simulink model "FBFunctions_Athira"  (R2018b)
settings: Solver=VariableStepAuto  StartTime=0.0  StopTime=10.0  RelTol=1e-3
values from neighbouring files (symbols this model uses):
  DIV = int32(25)    [setup.m]
  fractionalNumBits = 24    [setup.m]
  integerNumBits = 32    [setup.m]
  SUB = int32(23)    [setup.m]
undefined symbols (not defined in the file or in its folder): mask
libraries: library x94, hdlsllib x21, simulink x2
settings Model: Creator=hiterd  LastModifiedBy=jayakumarav
settings SFSimCC: SimUseLocalCustomCode=off
settings RTWCC: RTWUseLocalCustomCode=off

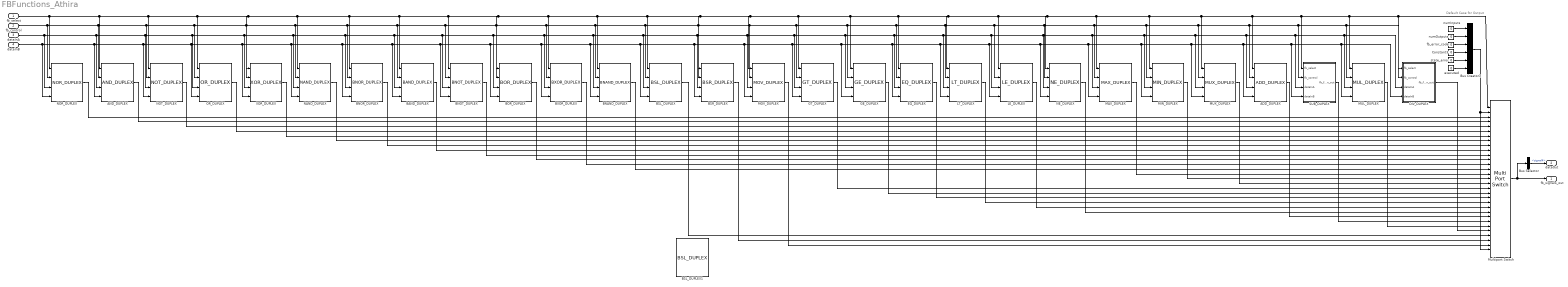
== system FBFunctions_Athira ==
  note: Default Case for Output
  fb_select : Inport  OutDataTypeStr=int32
  fb_control : Inport  Port=2  OutDataTypeStr=Bus: fb_control
  dataInA : Inport  Port=3  OutDataTypeStr=int32
  dataInB : Inport  Port=4  OutDataTypeStr=int32
  ADD_DUPLEX : library/ADD_DUPLEX  SystemSampleTime=-1  VariantControl=MUX_FB
  AND_DUPLEX : library/AND_DUPLEX  SystemSampleTime=-1  VariantControl=MUX_FB
  BAND_DUPLEX : library/BAND_DUPLEX  SystemSampleTime=-1  VariantControl=MUX_FB
  BNAND_DUPLEX : library/BNAND_DUPLEX  SystemSampleTime=-1  VariantControl=MUX_FB
  BNOR_DUPLEX : library/BNOR_DUPLEX  SystemSampleTime=-1  VariantControl=MUX_FB
  BNOT_DUPLEX : library/BNOT_DUPLEX  SystemSampleTime=-1  VariantControl=MUX_FB
  BOR_DUPLEX : library/BOR_DUPLEX  SystemSampleTime=-1  VariantControl=MUX_FB
  BSL_DUPLEX : library/BSL_DUPLEX  SystemSampleTime=-1  VariantControl=MUX_FB
  BSL_DUPLEX1 : library/BSL_DUPLEX  SystemSampleTime=-1  VariantControl=MUX_FB
  BSR_DUPLEX : library/BSR_DUPLEX  SystemSampleTime=-1  VariantControl=MUX_FB
  BXOR_DUPLEX : library/BXOR_DUPLEX  SystemSampleTime=-1  VariantControl=MUX_FB
  Bus Creator1 : BusCreator  Inputs=6  OutDataTypeStr=Bus: fb_functions_out
  Bus Selector : BusSelector  OutputSignals=signal4
  Constant3 : Constant  Value=0  OutDataTypeStr=int32  SampleTime=-1
  DIV_DUPLEX : Subsystem  AncestorBlock=library/DIV_DUPLEX  TreatAsAtomicUnit=on  VariantControl=MUX_FB
  EQ_DUPLEX : library/EQ_DUPLEX  SystemSampleTime=-1  VariantControl=MUX_FB
  GE_DUPLEX : library/GE_DUPLEX  SystemSampleTime=-1  VariantControl=MUX_FB
  GT_DUPLEX : library/GT_DUPLEX  SystemSampleTime=-1  VariantControl=MUX_FB
  LE_DUPLEX : library/LE_DUPLEX  SystemSampleTime=-1  VariantControl=MUX_FB
  LT_DUPLEX : library/LT_DUPLEX  SystemSampleTime=-1  VariantControl=MUX_FB
  MAX_DUPLEX : library/MAX_DUPLEX  SystemSampleTime=-1  VariantControl=MUX_FB
  MIN_DUPLEX : library/MIN_DUPLEX  SystemSampleTime=-1  VariantControl=MUX_FB
  MOV_DUPLEX : library/MOV_DUPLEX  SystemSampleTime=-1  VariantControl=MUX_FB
  MUL_DUPLEX : library/MUL_DUPLEX  SystemSampleTime=-1  VariantControl=MUX_FB
  MUX_DUPLEX : library/MUX_DUPLEX  SystemSampleTime=-1  VariantControl=MUX_FB
  Multiport Switch : MultiPortSwitch  DataPortOrder=Zero-based contiguous  Inputs=29  DataPortForDefault=Additional data port  zeroidx=on  OutDataTypeStr=Inherit: Inherit via back propagation
  NAND_DUPLEX : library/NAND_DUPLEX  SystemSampleTime=-1  VariantControl=MUX_FB
  NE_DUPLEX : library/NE_DUPLEX  SystemSampleTime=-1  VariantControl=MUX_FB
  NOR_DUPLEX : library/NOR_DUPLEX  SystemSampleTime=-1  VariantControl=MUX_FB
  NOT_DUPLEX : library/NOT_DUPLEX  SystemSampleTime=-1  VariantControl=MUX_FB
  OR_DUPLEX : library/OR_DUPLEX  SystemSampleTime=-1  VariantControl=MUX_FB
  SUB_DUPLEX : Subsystem  AncestorBlock=library/SUB_DUPLEX  TreatAsAtomicUnit=on  VariantControl=MUX_FB
  XOR_DUPLEX : library/XOR_DUPLEX  SystemSampleTime=-1  VariantControl=MUX_FB
  executed : Constant  Value=0  OutDataTypeStr=boolean  SampleTime=-1
  fb_error_code : Constant  Value=0  OutDataTypeStr=uint32  SampleTime=-1
  numInputs : Constant  Value=0  OutDataTypeStr=uint8  SampleTime=-1
  numOutputs : Constant  Value=0  OutDataTypeStr=uint8  SampleTime=-1
  state_error : Constant  Value=0  OutDataTypeStr=boolean  SampleTime=-1
  fb_signals_out : Outport  OutDataTypeStr=Bus: fb_functions_out
  dataOut : Outport  Port=2
  wires:
  Multiport Switch/1 -> fb_signals_out/1, Bus Selector/1
  Bus Selector/1 -> dataOut/1  "<signal4>"
  Bus Creator1/1 -> Multiport Switch/2, Multiport Switch/31
  numInputs/1 -> Bus Creator1/1
  executed/1 -> Bus Creator1/6
  state_error/1 -> Bus Creator1/5
  Constant3/1 -> Bus Creator1/4
  fb_error_code/1 -> Bus Creator1/3
  numOutputs/1 -> Bus Creator1/2
  fb_select/1 -> NOR_DUPLEX/1, AND_DUPLEX/1, NOT_DUPLEX/1, OR_DUPLEX/1, XOR_DUPLEX/1, NAND_DUPLEX/1, BNOR_DUPLEX/1, BAND_DUPLEX/1, BNOT_DUPLEX/1, BOR_DUPLEX/1, BXOR_DUPLEX/1, BNAND_DUPLEX/1, BSL_DUPLEX/1, BSR_DUPLEX/1, MOV_DUPLEX/1, GT_DUPLEX/1, GE_DUPLEX/1, EQ_DUPLEX/1, LT_DUPLEX/1, LE_DUPLEX/1, NE_DUPLEX/1, MAX_DUPLEX/1, MIN_DUPLEX/1, MUX_DUPLEX/1, ADD_DUPLEX/1, SUB_DUPLEX/1(fb_select), MUL_DUPLEX/1, DIV_DUPLEX/1(fb_select), Multiport Switch/1
  fb_control/1 -> NOR_DUPLEX/2, AND_DUPLEX/2, NOT_DUPLEX/2, OR_DUPLEX/2, XOR_DUPLEX/2, NAND_DUPLEX/2, BNOR_DUPLEX/2, BAND_DUPLEX/2, BNOT_DUPLEX/2, BOR_DUPLEX/2, BXOR_DUPLEX/2, BNAND_DUPLEX/2, BSL_DUPLEX/2, BSR_DUPLEX/2, MOV_DUPLEX/2, GT_DUPLEX/2, GE_DUPLEX/2, EQ_DUPLEX/2, LT_DUPLEX/2, LE_DUPLEX/2, NE_DUPLEX/2, MAX_DUPLEX/2, MIN_DUPLEX/2, MUX_DUPLEX/2, ADD_DUPLEX/2, SUB_DUPLEX/2(fb_control), MUL_DUPLEX/2, DIV_DUPLEX/2(fb_control)
  dataInA/1 -> NOR_DUPLEX/3, AND_DUPLEX/3, NOT_DUPLEX/3, OR_DUPLEX/3, XOR_DUPLEX/3, NAND_DUPLEX/3, BNOR_DUPLEX/3, BAND_DUPLEX/3, BNOT_DUPLEX/3, BOR_DUPLEX/3, BXOR_DUPLEX/3, BNAND_DUPLEX/3, BSL_DUPLEX/3, BSR_DUPLEX/3, MOV_DUPLEX/3, GT_DUPLEX/3, GE_DUPLEX/3, EQ_DUPLEX/3, LT_DUPLEX/3, LE_DUPLEX/3, NE_DUPLEX/3, MAX_DUPLEX/3, MIN_DUPLEX/3, MUX_DUPLEX/3, ADD_DUPLEX/3, SUB_DUPLEX/3(dataInA), MUL_DUPLEX/3, DIV_DUPLEX/3(dataInA)
  dataInB/1 -> NOR_DUPLEX/4, AND_DUPLEX/4, NOT_DUPLEX/4, OR_DUPLEX/4, XOR_DUPLEX/4, NAND_DUPLEX/4, BNOR_DUPLEX/4, BAND_DUPLEX/4, BNOT_DUPLEX/4, BOR_DUPLEX/4, BXOR_DUPLEX/4, BNAND_DUPLEX/4, BSL_DUPLEX/4, BSR_DUPLEX/4, MOV_DUPLEX/4, GT_DUPLEX/4, GE_DUPLEX/4, EQ_DUPLEX/4, LT_DUPLEX/4, LE_DUPLEX/4, NE_DUPLEX/4, MAX_DUPLEX/4, MIN_DUPLEX/4, MUX_DUPLEX/4, ADD_DUPLEX/4, SUB_DUPLEX/4(dataInB), MUL_DUPLEX/4, DIV_DUPLEX/4(dataInB)
  DIV_DUPLEX/1(fb_function_out) -> Multiport Switch/27
  MUL_DUPLEX/1 -> Multiport Switch/26
  SUB_DUPLEX/1(fb_function_out) -> Multiport Switch/25
  ADD_DUPLEX/1 -> Multiport Switch/24
  MUX_DUPLEX/1 -> Multiport Switch/17
  MIN_DUPLEX/1 -> Multiport Switch/16
  MAX_DUPLEX/1 -> Multiport Switch/15
  NE_DUPLEX/1 -> Multiport Switch/23
  LE_DUPLEX/1 -> Multiport Switch/22
  LT_DUPLEX/1 -> Multiport Switch/21
  EQ_DUPLEX/1 -> Multiport Switch/20
  GE_DUPLEX/1 -> Multiport Switch/19
  GT_DUPLEX/1 -> Multiport Switch/18
  MOV_DUPLEX/1 -> Multiport Switch/30
  BSR_DUPLEX/1 -> Multiport Switch/29
  BSL_DUPLEX/1 -> Multiport Switch/28
  BNAND_DUPLEX/1 -> Multiport Switch/14
  BXOR_DUPLEX/1 -> Multiport Switch/13
  BOR_DUPLEX/1 -> Multiport Switch/12
  BNOT_DUPLEX/1 -> Multiport Switch/11
  BAND_DUPLEX/1 -> Multiport Switch/10
  BNOR_DUPLEX/1 -> Multiport Switch/9
  NAND_DUPLEX/1 -> Multiport Switch/8
  XOR_DUPLEX/1 -> Multiport Switch/7
  OR_DUPLEX/1 -> Multiport Switch/6
  NOT_DUPLEX/1 -> Multiport Switch/5
  AND_DUPLEX/1 -> Multiport Switch/4
  NOR_DUPLEX/1 -> Multiport Switch/3

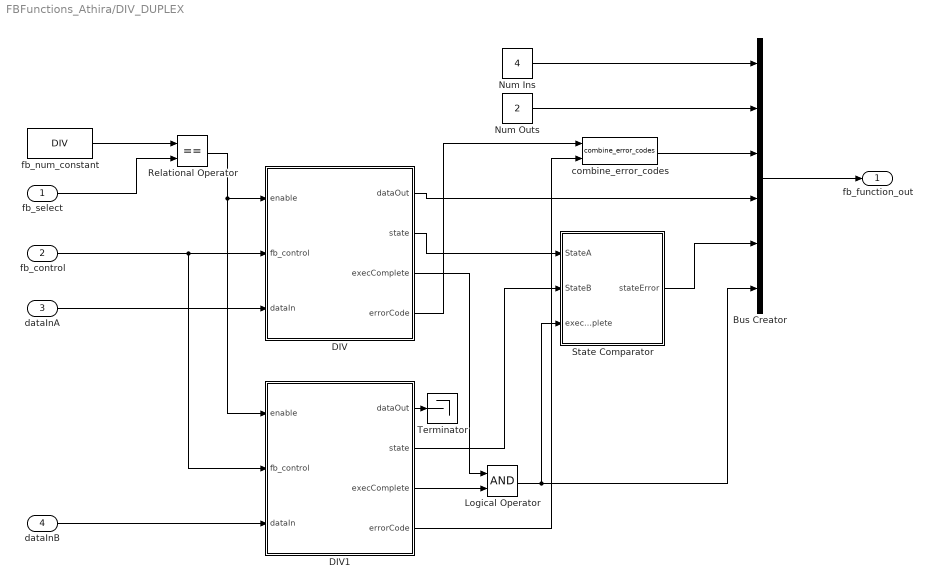
== system FBFunctions_Athira/DIV_DUPLEX ==
  fb_select : Inport  RequirementInfo={} %GIDa_689071d9_cee7_4e2c_b7c4_80b6ba1221c0
  fb_control : Inport  RequirementInfo={} %GIDa_11a08c44_a509_4d4e_9977_4ee3096f5a96  Port=2  OutDataTypeStr=Bus: fb_control
  dataInA : Inport  RequirementInfo={} %GIDa_676e53ea_4d29_43e9_b26a_819a8a097af1  Port=3
  dataInB : Inport  RequirementInfo={} %GIDa_576eb6ee_66f4_422a_ac92_7848b70f5695  Port=4
  Bus Creator : BusCreator  RequirementInfo={} %GIDa_1e0b0d89_1a78_4d77_bc56_e7844c63960f  Inputs=6  OutDataTypeStr=Bus: fb_functions_out
  DIV : Subsystem  AncestorBlock=library/DIV
  DIV1 : Subsystem  AncestorBlock=library/DIV
  Logical Operator : Logic  RequirementInfo={} %GIDa_310cbc44_5d27_4b1d_b2cc_f35da33db360  AllPortsSameDT=off  OutDataTypeStr=boolean
  Num Ins : Constant  RequirementInfo={} %GIDa_5073ddfd_09c4_48ad_98ad_a17e52741fae  Value=4  OutDataTypeStr=Inherit: Inherit via back propagation
  Num Outs : Constant  RequirementInfo={} %GIDa_9f8fac5a_a9cf_4741_a97b_37f3b3ddc735  Value=2  OutDataTypeStr=Inherit: Inherit via back propagation
  Relational Operator : RelationalOperator  RequirementInfo={} %GIDa_ab00c8df_eece_4939_b262_293eca2149e3  Operator===  OutDataTypeStr=boolean  RndMeth=Nearest
  State Comparator : Subsystem  RequirementInfo={} %GIDa_7d81c358_2c1e_4ce4_a0ef_1c9d194247af
  Terminator : Terminator
      settings: RequirementInfo={} %GIDa_30e5f69c_fd7b_4ac2_95db_4cee4b8383fb
  combine_error_codes : library/combine_error_codes  SystemSampleTime=-1
  fb_num_constant : Constant  RequirementInfo={} %GIDa_c891fb26_8c71_4395_9cd7_0c55d875d13d  Value=DIV
  fb_function_out : Outport  RequirementInfo={} %GIDa_ad45d925_6996_4e52_8ffb_8b13a833d5f7  OutDataTypeStr=Bus: fb_functions_out
  wires:
  DIV1/4(errorCode) -> combine_error_codes/2
  combine_error_codes/1 -> Bus Creator/3
  Relational Operator/1 -> DIV/1(enable), DIV1/1(enable)
  DIV/1(dataOut) -> Bus Creator/4
  Bus Creator/1 -> fb_function_out/1
  fb_control/1 -> DIV/2(fb_control), DIV1/2(fb_control)
  dataInB/1 -> DIV1/3(dataIn)
  fb_select/1 -> Relational Operator/2
  fb_num_constant/1 -> Relational Operator/1
  State Comparator/1(stateError) -> Bus Creator/5
  DIV/4(errorCode) -> combine_error_codes/1
  DIV1/1(dataOut) -> Terminator/1
  DIV1/3(execComplete) -> Logical Operator/2
  DIV/3(execComplete) -> Logical Operator/1
  Logical Operator/1 -> State Comparator/3(execComplete), Bus Creator/6
  Num Outs/1 -> Bus Creator/2
  DIV1/2(state) -> State Comparator/2(StateB)
  DIV/2(state) -> State Comparator/1(StateA)
  dataInA/1 -> DIV/3(dataIn)
  Num Ins/1 -> Bus Creator/1

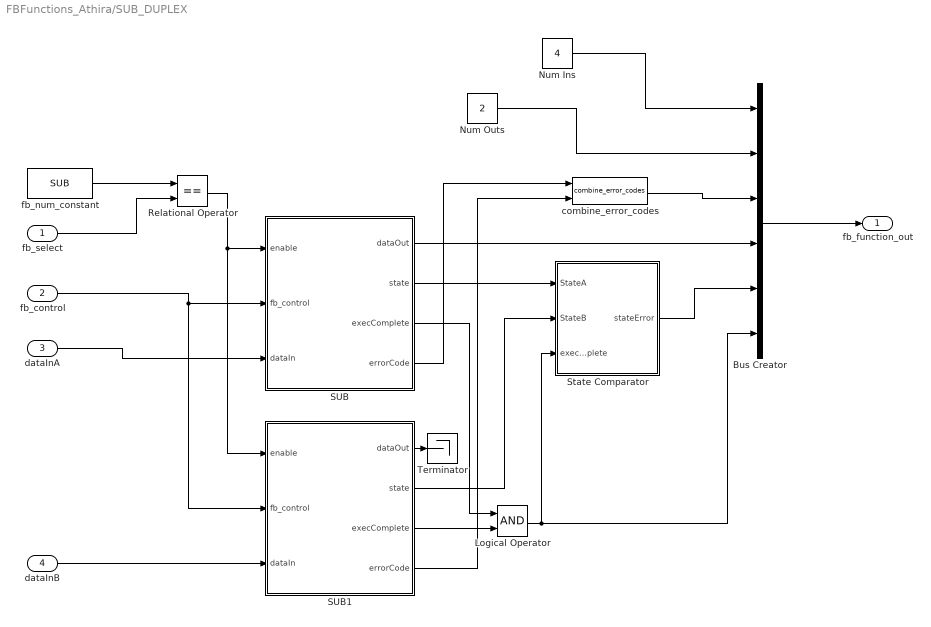
== system FBFunctions_Athira/SUB_DUPLEX ==
  fb_select : Inport  RequirementInfo={} %GIDa_689071d9_cee7_4e2c_b7c4_80b6ba1221c0
  fb_control : Inport  RequirementInfo={} %GIDa_11a08c44_a509_4d4e_9977_4ee3096f5a96  Port=2  OutDataTypeStr=Bus: fb_control
  dataInA : Inport  RequirementInfo={} %GIDa_676e53ea_4d29_43e9_b26a_819a8a097af1  Port=3
  dataInB : Inport  RequirementInfo={} %GIDa_576eb6ee_66f4_422a_ac92_7848b70f5695  Port=4
  Bus Creator : BusCreator  RequirementInfo={} %GIDa_1e0b0d89_1a78_4d77_bc56_e7844c63960f  Inputs=6  OutDataTypeStr=Bus: fb_functions_out
  Logical Operator : Logic  RequirementInfo={} %GIDa_310cbc44_5d27_4b1d_b2cc_f35da33db360  AllPortsSameDT=off  OutDataTypeStr=boolean
  Num Ins : Constant  RequirementInfo={} %GIDa_5073ddfd_09c4_48ad_98ad_a17e52741fae  Value=4  OutDataTypeStr=Inherit: Inherit via back propagation
  Num Outs : Constant  RequirementInfo={} %GIDa_9f8fac5a_a9cf_4741_a97b_37f3b3ddc735  Value=2  OutDataTypeStr=Inherit: Inherit via back propagation
  Relational Operator : RelationalOperator  RequirementInfo={} %GIDa_ab00c8df_eece_4939_b262_293eca2149e3  Operator===  OutDataTypeStr=boolean  RndMeth=Nearest
  SUB : Subsystem  AncestorBlock=library/SUB
  SUB1 : Subsystem  AncestorBlock=library/SUB
  State Comparator : Subsystem  RequirementInfo={} %GIDa_7d81c358_2c1e_4ce4_a0ef_1c9d194247af
  Terminator : Terminator
      settings: RequirementInfo={} %GIDa_30e5f69c_fd7b_4ac2_95db_4cee4b8383fb
  combine_error_codes : library/combine_error_codes  SystemSampleTime=-1
  fb_num_constant : Constant  RequirementInfo={} %GIDa_c891fb26_8c71_4395_9cd7_0c55d875d13d  Value=SUB
  fb_function_out : Outport  RequirementInfo={} %GIDa_ad45d925_6996_4e52_8ffb_8b13a833d5f7  OutDataTypeStr=Bus: fb_functions_out
  wires:
  SUB1/4(errorCode) -> combine_error_codes/2
  combine_error_codes/1 -> Bus Creator/3
  Relational Operator/1 -> SUB/1(enable), SUB1/1(enable)
  SUB/1(dataOut) -> Bus Creator/4
  Bus Creator/1 -> fb_function_out/1
  fb_control/1 -> SUB/2(fb_control), SUB1/2(fb_control)
  dataInB/1 -> SUB1/3(dataIn)
  fb_select/1 -> Relational Operator/2
  fb_num_constant/1 -> Relational Operator/1
  State Comparator/1(stateError) -> Bus Creator/5
  SUB/4(errorCode) -> combine_error_codes/1
  SUB1/1(dataOut) -> Terminator/1
  SUB1/3(execComplete) -> Logical Operator/2
  SUB/3(execComplete) -> Logical Operator/1
  Logical Operator/1 -> State Comparator/3(execComplete), Bus Creator/6
  Num Outs/1 -> Bus Creator/2
  SUB1/2(state) -> State Comparator/2(StateB)
  SUB/2(state) -> State Comparator/1(StateA)
  dataInA/1 -> SUB/3(dataIn)
  Num Ins/1 -> Bus Creator/1

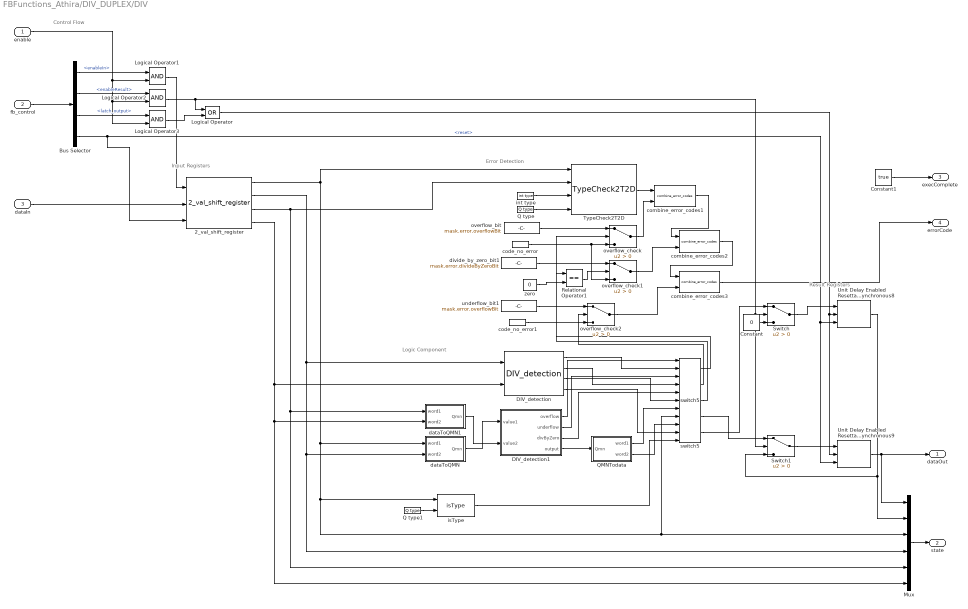
== system FBFunctions_Athira/DIV_DUPLEX/DIV ==
  note: Logic Component
  note: Input Registers
  note: Control Flow
  note: Result Registers
  note: Error Detection
  enable : Inport  OutDataTypeStr=boolean
  fb_control : Inport  Port=2  OutDataTypeStr=Bus: fb_control
  dataIn : Inport  Port=3  OutDataTypeStr=int32
  2_val_shift_register : library/2_val_shift_register  SystemSampleTime=-1
  Bus Selector : BusSelector  OutputSignals=enableIn,enableResult,latch_output,reset
  Constant : Constant  Value=0  OutDataTypeStr=int32
  Constant1 : Constant  Value=true  SampleTime=-1
  DIV_detection : library/DIV_detection  SystemSampleTime=-1
  DIV_detection1 : Subsystem  AncestorBlock=library/DIV_detection
  Logical Operator : Logic  Operator=OR  AllPortsSameDT=off  OutDataTypeStr=boolean
  Logical Operator1 : Logic  AllPortsSameDT=off  OutDataTypeStr=boolean
  Logical Operator2 : Logic  AllPortsSameDT=off  OutDataTypeStr=boolean
  Logical Operator3 : Logic  AllPortsSameDT=off  OutDataTypeStr=boolean
  Mux : Mux  Inputs=6
  Q type : library/Q type  SystemSampleTime=-1
  Q type1 : library/Q type  SystemSampleTime=-1
  QMNTodata : Subsystem  AncestorBlock=library/QMNTodata
  Relational Operator1 : RelationalOperator  Operator===  OutDataTypeStr=boolean  RndMeth=Nearest
  Switch : Switch  Criteria=u2 > Threshold
  Switch1 : Switch  Criteria=u2 > Threshold
  TypeCheck2T2D : library/TypeCheck2T2D  SystemSampleTime=-1
  Unit Delay Enabled Resettable Synchronous8 : hdlsllib/Discrete/Unit Delay Enabled Resettable Synchronous  InitialCondition=0.0  SampleTime=-1
      settings: SourceProductName=HDL Coder  SourceProductBaseCode=HD
  Unit Delay Enabled Resettable Synchronous9 : hdlsllib/Discrete/Unit Delay Enabled Resettable Synchronous  InitialCondition=0.0  SampleTime=-1
      settings: SourceProductName=HDL Coder  SourceProductBaseCode=HD
  code_no_error : library/code_no_error  SystemSampleTime=-1
  code_no_error1 : library/code_no_error  SystemSampleTime=-1
  combine_error_codes1 : library/combine_error_codes  SystemSampleTime=-1
  combine_error_codes2 : library/combine_error_codes  SystemSampleTime=-1
  combine_error_codes3 : library/combine_error_codes  SystemSampleTime=-1
  dataToQMN : Subsystem  AncestorBlock=library/dataToQMN
  dataToQMN1 : Subsystem  AncestorBlock=library/dataToQMN
  divide_by_zero_bit1 : Constant  Value=mask.error.divideByZeroBit  SampleTime=-1
  int type : library/int type  SystemSampleTime=-1
  isType : library/isType  SystemSampleTime=-1
  overflow_bit : Constant  Value=mask.error.overflowBit  SampleTime=-1
  overflow_check : Switch  Criteria=u2 > Threshold
  overflow_check1 : Switch  Criteria=u2 > Threshold
  overflow_check2 : Switch  Criteria=u2 > Threshold
  switch5 : library/switch5  SystemSampleTime=-1
  underflow_bit1 : Constant  Value=mask.error.overflowBit  SampleTime=-1
  zero : Constant  Value=0  SampleTime=-1
  dataOut : Outport
  state : Outport  Port=2
  execComplete : Outport  Port=3  OutDataTypeStr=boolean  PortDimensions=1
  errorCode : Outport  Port=4  PortDimensions=1
  wires:
  dataToQMN1/1(Qmn) -> DIV_detection1/2(value2)
  dataToQMN/1(Qmn) -> DIV_detection1/1(value1)
  combine_error_codes2/1 -> combine_error_codes3/1
  overflow_check2/1 -> combine_error_codes3/2
  code_no_error1/1 -> overflow_check2/3
  underflow_bit1/1 -> overflow_check2/1
  switch5/3 -> Relational Operator1/1
  DIV_detection1/3(divByZero) -> switch5/5
  DIV_detection/3 -> switch5/6
  switch5/1 -> overflow_check/2
  DIV_detection1/1(overflow) -> switch5/1
  QMNTodata/2(word2) -> switch5/9
  DIV_detection/1 -> switch5/2
  isType/1 -> switch5/11
  2_val_shift_register/2 -> Mux/4, dataToQMN/2(word2), DIV_detection/1
  DIV_detection/2 -> switch5/4
  Q type1/1 -> isType/2
  2_val_shift_register/1 -> TypeCheck2T2D/1, isType/1, Mux/3, switch5/8, dataToQMN/1(word1)
  switch5/2 -> overflow_check2/2
  DIV_detection1/2(underflow) -> switch5/3
  switch5/5 -> Switch/1
  DIV_detection1/4(output) -> QMNTodata/1(Qmn)
  2_val_shift_register/4 -> Mux/6, dataToQMN1/2(word2), DIV_detection/2
  switch5/4 -> Switch1/1
  2_val_shift_register/3 -> Mux/5, dataToQMN1/1(word1), TypeCheck2T2D/2
  QMNTodata/1(word1) -> switch5/7
  DIV_detection/4 -> switch5/10
  overflow_check1/1 -> combine_error_codes2/2
  combine_error_codes1/1 -> combine_error_codes2/1
  zero/1 -> Relational Operator1/2
  Relational Operator1/1 -> overflow_check1/2
  divide_by_zero_bit1/1 -> overflow_check1/1
  Unit Delay Enabled Resettable Synchronous8/1 -> Switch1/3, Mux/2
  Mux/1 -> state/1
  Unit Delay Enabled Resettable Synchronous9/1 -> dataOut/1, Mux/1
  Switch1/1 -> Unit Delay Enabled Resettable Synchronous9/1
  Logical Operator2/1 -> Logical Operator/1, Switch/2, Switch1/2
  Switch/1 -> Unit Delay Enabled Resettable Synchronous8/1
  Logical Operator/1 -> Unit Delay Enabled Resettable Synchronous9/2, Unit Delay Enabled Resettable Synchronous8/2
  Logical Operator3/1 -> Logical Operator/2
  Bus Selector/4 -> Unit Delay Enabled Resettable Synchronous9/3, Unit Delay Enabled Resettable Synchronous8/3, 2_val_shift_register/3  "<reset>"
  Logical Operator1/1 -> 2_val_shift_register/1
  dataIn/1 -> 2_val_shift_register/2
  Constant/1 -> Switch/3
  Constant1/1 -> execComplete/1
  fb_control/1 -> Bus Selector/1
  Bus Selector/3 -> Logical Operator3/1  "<latch_output>"
  Bus Selector/1 -> Logical Operator1/1  "<enableIn>"
  Bus Selector/2 -> Logical Operator2/1  "<enableResult>"
  enable/1 -> Logical Operator2/2, Logical Operator3/2, Logical Operator1/2
  TypeCheck2T2D/1 -> combine_error_codes1/1
  Q type/1 -> TypeCheck2T2D/4
  int type/1 -> TypeCheck2T2D/3
  combine_error_codes3/1 -> errorCode/1
  overflow_bit/1 -> overflow_check/1
  code_no_error/1 -> overflow_check/3, overflow_check1/3
  overflow_check/1 -> combine_error_codes1/2

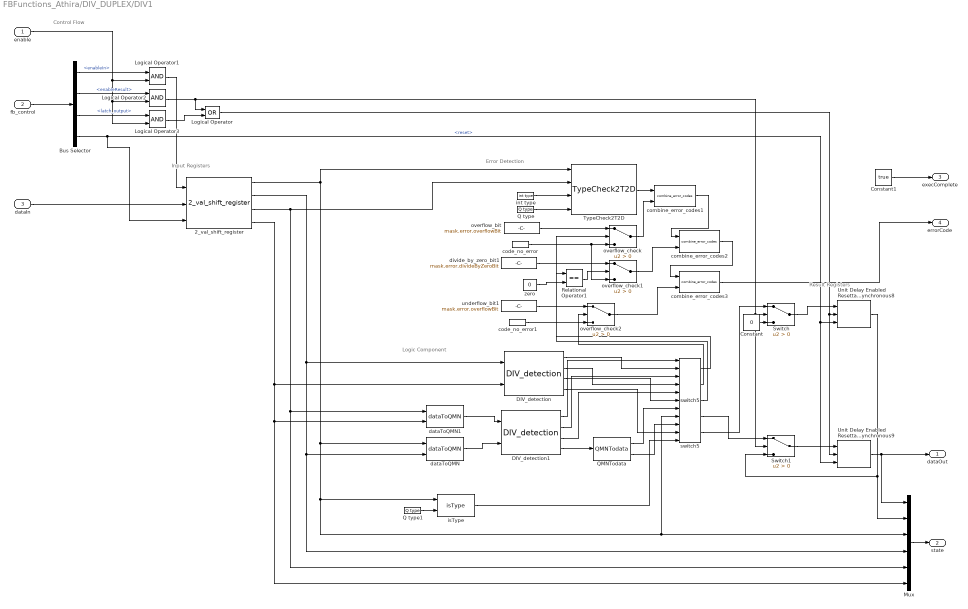
== system FBFunctions_Athira/DIV_DUPLEX/DIV1 ==
  note: Logic Component
  note: Input Registers
  note: Control Flow
  note: Result Registers
  note: Error Detection
  enable : Inport  OutDataTypeStr=boolean
  fb_control : Inport  Port=2  OutDataTypeStr=Bus: fb_control
  dataIn : Inport  Port=3  OutDataTypeStr=int32
  2_val_shift_register : library/2_val_shift_register  SystemSampleTime=-1
  Bus Selector : BusSelector  OutputSignals=enableIn,enableResult,latch_output,reset
  Constant : Constant  Value=0  OutDataTypeStr=int32
  Constant1 : Constant  Value=true  SampleTime=-1
  DIV_detection : library/DIV_detection  SystemSampleTime=-1
  DIV_detection1 : library/DIV_detection  SystemSampleTime=-1
  Logical Operator : Logic  Operator=OR  AllPortsSameDT=off  OutDataTypeStr=boolean
  Logical Operator1 : Logic  AllPortsSameDT=off  OutDataTypeStr=boolean
  Logical Operator2 : Logic  AllPortsSameDT=off  OutDataTypeStr=boolean
  Logical Operator3 : Logic  AllPortsSameDT=off  OutDataTypeStr=boolean
  Mux : Mux  Inputs=6
  Q type : library/Q type  SystemSampleTime=-1
  Q type1 : library/Q type  SystemSampleTime=-1
  QMNTodata : library/QMNTodata  SystemSampleTime=-1
      link override fractional2: lidx=31  ridx=24
  Relational Operator1 : RelationalOperator  Operator===  OutDataTypeStr=boolean  RndMeth=Nearest
  Switch : Switch  Criteria=u2 > Threshold
  Switch1 : Switch  Criteria=u2 > Threshold
  TypeCheck2T2D : library/TypeCheck2T2D  SystemSampleTime=-1
  Unit Delay Enabled Resettable Synchronous8 : hdlsllib/Discrete/Unit Delay Enabled Resettable Synchronous  InitialCondition=0.0  SampleTime=-1
      settings: SourceProductName=HDL Coder  SourceProductBaseCode=HD
  Unit Delay Enabled Resettable Synchronous9 : hdlsllib/Discrete/Unit Delay Enabled Resettable Synchronous  InitialCondition=0.0  SampleTime=-1
      settings: SourceProductName=HDL Coder  SourceProductBaseCode=HD
  code_no_error : library/code_no_error  SystemSampleTime=-1
  code_no_error1 : library/code_no_error  SystemSampleTime=-1
  combine_error_codes1 : library/combine_error_codes  SystemSampleTime=-1
  combine_error_codes2 : library/combine_error_codes  SystemSampleTime=-1
  combine_error_codes3 : library/combine_error_codes  SystemSampleTime=-1
  dataToQMN : library/dataToQMN  SystemSampleTime=-1
  dataToQMN1 : library/dataToQMN  SystemSampleTime=-1
  divide_by_zero_bit1 : Constant  Value=mask.error.divideByZeroBit  SampleTime=-1
  int type : library/int type  SystemSampleTime=-1
  isType : library/isType  SystemSampleTime=-1
  overflow_bit : Constant  Value=mask.error.overflowBit  SampleTime=-1
  overflow_check : Switch  Criteria=u2 > Threshold
  overflow_check1 : Switch  Criteria=u2 > Threshold
  overflow_check2 : Switch  Criteria=u2 > Threshold
  switch5 : library/switch5  SystemSampleTime=-1
  underflow_bit1 : Constant  Value=mask.error.overflowBit  SampleTime=-1
  zero : Constant  Value=0  SampleTime=-1
  dataOut : Outport
  state : Outport  Port=2
  execComplete : Outport  Port=3  OutDataTypeStr=boolean  PortDimensions=1
  errorCode : Outport  Port=4  PortDimensions=1
  wires:
  combine_error_codes2/1 -> combine_error_codes3/1
  overflow_check2/1 -> combine_error_codes3/2
  code_no_error1/1 -> overflow_check2/3
  underflow_bit1/1 -> overflow_check2/1
  switch5/3 -> Relational Operator1/1
  DIV_detection1/3 -> switch5/5
  DIV_detection/3 -> switch5/6
  switch5/1 -> overflow_check/2
  DIV_detection1/1 -> switch5/1
  QMNTodata/2 -> switch5/9
  DIV_detection/1 -> switch5/2
  isType/1 -> switch5/11
  2_val_shift_register/2 -> Mux/4, dataToQMN/2, DIV_detection/1
  DIV_detection/2 -> switch5/4
  Q type1/1 -> isType/2
  2_val_shift_register/1 -> TypeCheck2T2D/1, isType/1, Mux/3, switch5/8, dataToQMN/1
  switch5/2 -> overflow_check2/2
  dataToQMN1/1 -> DIV_detection1/1
  DIV_detection1/2 -> switch5/3
  switch5/5 -> Switch/1
  DIV_detection1/4 -> QMNTodata/1
  2_val_shift_register/4 -> Mux/6, dataToQMN1/2, DIV_detection/2
  switch5/4 -> Switch1/1
  2_val_shift_register/3 -> Mux/5, dataToQMN1/1, TypeCheck2T2D/2
  QMNTodata/1 -> switch5/7
  DIV_detection/4 -> switch5/10
  dataToQMN/1 -> DIV_detection1/2
  overflow_check1/1 -> combine_error_codes2/2
  combine_error_codes1/1 -> combine_error_codes2/1
  zero/1 -> Relational Operator1/2
  Relational Operator1/1 -> overflow_check1/2
  divide_by_zero_bit1/1 -> overflow_check1/1
  Unit Delay Enabled Resettable Synchronous8/1 -> Switch1/3, Mux/2
  Mux/1 -> state/1
  Unit Delay Enabled Resettable Synchronous9/1 -> dataOut/1, Mux/1
  Switch1/1 -> Unit Delay Enabled Resettable Synchronous9/1
  Logical Operator2/1 -> Logical Operator/1, Switch/2, Switch1/2
  Switch/1 -> Unit Delay Enabled Resettable Synchronous8/1
  Logical Operator/1 -> Unit Delay Enabled Resettable Synchronous9/2, Unit Delay Enabled Resettable Synchronous8/2
  Logical Operator3/1 -> Logical Operator/2
  Bus Selector/4 -> Unit Delay Enabled Resettable Synchronous9/3, Unit Delay Enabled Resettable Synchronous8/3, 2_val_shift_register/3  "<reset>"
  Logical Operator1/1 -> 2_val_shift_register/1
  dataIn/1 -> 2_val_shift_register/2
  Constant/1 -> Switch/3
  Constant1/1 -> execComplete/1
  fb_control/1 -> Bus Selector/1
  Bus Selector/3 -> Logical Operator3/1  "<latch_output>"
  Bus Selector/1 -> Logical Operator1/1  "<enableIn>"
  Bus Selector/2 -> Logical Operator2/1  "<enableResult>"
  enable/1 -> Logical Operator2/2, Logical Operator3/2, Logical Operator1/2
  TypeCheck2T2D/1 -> combine_error_codes1/1
  Q type/1 -> TypeCheck2T2D/4
  int type/1 -> TypeCheck2T2D/3
  combine_error_codes3/1 -> errorCode/1
  overflow_bit/1 -> overflow_check/1
  code_no_error/1 -> overflow_check/3, overflow_check1/3
  overflow_check/1 -> combine_error_codes1/2

== system FBFunctions_Athira/DIV_DUPLEX/State Comparator ==
  StateA : Inport  RequirementInfo={} %GIDa_850ba5fb_bec6_40a7_bff2_e88e25707b72
  StateB : Inport  RequirementInfo={} %GIDa_31d9701c_a33d_4ba1_b762_d6eba5e746ea  Port=2
  execComplete : Inport  RequirementInfo={} %GIDa_6900b5eb_6e34_4b5c_ab46_3bf84fbb4fde  Port=3
  Compare To Zero : simulink/Logic and Bit Operations/Compare To Zero  relop=>  OutDataTypeStr=boolean
  Constant1 : Constant  RequirementInfo={} %GIDa_e6dc7871_9460_47b7_844d_fe346f2ff008  Value=false  SampleTime=-1
  Relational Operator : RelationalOperator  RequirementInfo={} %GIDa_bc019a10_ee56_46ec_8d92_4f9a7b675e24  Operator=~=  OutDataTypeStr=boolean  RndMeth=Simplest
  Sum of Elements : Sum  RequirementInfo={} %GIDa_4b7ccedc_73e5_4206_ba44_2065d6a036fb  Inputs=+
  Switch1 : Switch  RequirementInfo={} %GIDa_a5db4cb6_7e1e_4dca_a520_beca643cf818  Criteria=u2 > Threshold
  stateError : Outport  RequirementInfo={} %GIDa_debaf768_048f_4ef3_86a7_3d4e6bd99aa3
  wires:
  Compare To Zero/1 -> Switch1/1
  Sum of Elements/1 -> Compare To Zero/1
  Relational Operator/1 -> Sum of Elements/1
  Switch1/1 -> stateError/1
  execComplete/1 -> Switch1/2
  Constant1/1 -> Switch1/3
  StateB/1 -> Relational Operator/2
  StateA/1 -> Relational Operator/1

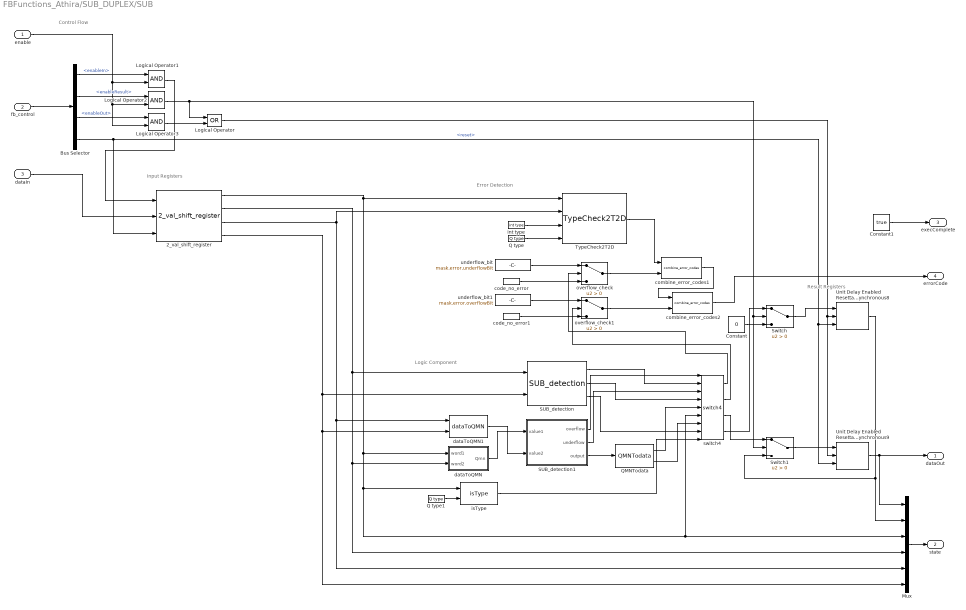
== system FBFunctions_Athira/SUB_DUPLEX/SUB ==
  note: Logic Component
  note: Input Registers
  note: Control Flow
  note: Error Detection
  note: Result Registers
  enable : Inport  OutDataTypeStr=boolean
  fb_control : Inport  Port=2  OutDataTypeStr=Bus: fb_control
  dataIn : Inport  Port=3  OutDataTypeStr=int32
  2_val_shift_register : library/2_val_shift_register  SystemSampleTime=-1
  Bus Selector : BusSelector  OutputSignals=enableIn,enableResult,enableOut,reset
  Constant : Constant  Value=0  OutDataTypeStr=int32
  Constant1 : Constant  Value=true  SampleTime=-1
  Logical Operator : Logic  Operator=OR  AllPortsSameDT=off  OutDataTypeStr=boolean
  Logical Operator1 : Logic  AllPortsSameDT=off  OutDataTypeStr=boolean
  Logical Operator2 : Logic  AllPortsSameDT=off  OutDataTypeStr=boolean
  Logical Operator3 : Logic  AllPortsSameDT=off  OutDataTypeStr=boolean
  Mux : Mux  Inputs=6
  Q type : library/Q type  SystemSampleTime=-1
  Q type1 : library/Q type  SystemSampleTime=-1
  QMNTodata : library/QMNTodata  SystemSampleTime=-1
      link override fractional2: lidx=31  ridx=24
  SUB_detection : library/SUB_detection  SystemSampleTime=-1
  SUB_detection1 : Subsystem  AncestorBlock=library/SUB_detection
  Switch : Switch  Criteria=u2 > Threshold
  Switch1 : Switch  Criteria=u2 > Threshold
  TypeCheck2T2D : library/TypeCheck2T2D  SystemSampleTime=-1
  Unit Delay Enabled Resettable Synchronous8 : hdlsllib/Discrete/Unit Delay Enabled Resettable Synchronous  InitialCondition=0.0  SampleTime=-1
      settings: SourceProductName=HDL Coder  SourceProductBaseCode=HD
  Unit Delay Enabled Resettable Synchronous9 : hdlsllib/Discrete/Unit Delay Enabled Resettable Synchronous  InitialCondition=0.0  SampleTime=-1
      settings: SourceProductName=HDL Coder  SourceProductBaseCode=HD
  code_no_error : library/code_no_error  SystemSampleTime=-1
  code_no_error1 : library/code_no_error  SystemSampleTime=-1
  combine_error_codes1 : library/combine_error_codes  SystemSampleTime=-1
  combine_error_codes2 : library/combine_error_codes  SystemSampleTime=-1
  dataToQMN : Subsystem  AncestorBlock=library/dataToQMN
  dataToQMN1 : library/dataToQMN  SystemSampleTime=-1
  int type : library/int type  SystemSampleTime=-1
  isType : library/isType  SystemSampleTime=-1
  overflow_check : Switch  Criteria=u2 > Threshold
  overflow_check1 : Switch  Criteria=u2 > Threshold
  switch4 : library/switch4  SystemSampleTime=-1
  underflow_bit : Constant  Value=mask.error.underflowBit  SampleTime=-1
  underflow_bit1 : Constant  Value=mask.error.overflowBit  SampleTime=-1
  dataOut : Outport
  state : Outport  Port=2
  execComplete : Outport  Port=3  OutDataTypeStr=boolean  PortDimensions=1
  errorCode : Outport  Port=4  PortDimensions=1
  wires:
  dataToQMN/1(Qmn) -> SUB_detection1/1(value1)
  dataToQMN1/1 -> SUB_detection1/2(value2)
  switch4/1 -> overflow_check/2
  SUB_detection1/1(overflow) -> switch4/1
  QMNTodata/2 -> switch4/7
  2_val_shift_register/1 -> isType/1, Mux/3, switch4/6, dataToQMN/1(word1), TypeCheck2T2D/1
  SUB_detection/1 -> switch4/2
  isType/1 -> switch4/9
  SUB_detection/2 -> switch4/4
  Q type1/1 -> isType/2
  switch4/2 -> overflow_check1/2
  2_val_shift_register/4 -> Mux/6, dataToQMN1/2, SUB_detection/2
  SUB_detection1/2(underflow) -> switch4/3
  switch4/4 -> Switch/1
  SUB_detection1/3(output) -> QMNTodata/1
  switch4/3 -> Switch1/1
  2_val_shift_register/3 -> Mux/5, dataToQMN1/1, TypeCheck2T2D/2
  2_val_shift_register/2 -> Mux/4, dataToQMN/2(word2), SUB_detection/1
  QMNTodata/1 -> switch4/5
  SUB_detection/3 -> switch4/8
  combine_error_codes1/1 -> combine_error_codes2/1
  underflow_bit1/1 -> overflow_check1/1
  code_no_error1/1 -> overflow_check1/3
  overflow_check1/1 -> combine_error_codes2/2
  overflow_check/1 -> combine_error_codes1/2
  code_no_error/1 -> overflow_check/3
  underflow_bit/1 -> overflow_check/1
  combine_error_codes2/1 -> errorCode/1
  int type/1 -> TypeCheck2T2D/3
  Q type/1 -> TypeCheck2T2D/4
  TypeCheck2T2D/1 -> combine_error_codes1/1
  enable/1 -> Logical Operator1/2, Logical Operator3/2, Logical Operator2/2
  Bus Selector/2 -> Logical Operator2/1  "<enableResult>"
  Bus Selector/1 -> Logical Operator1/1  "<enableIn>"
  Bus Selector/3 -> Logical Operator3/1  "<enableOut>"
  fb_control/1 -> Bus Selector/1
  Constant1/1 -> execComplete/1
  Constant/1 -> Switch/3
  dataIn/1 -> 2_val_shift_register/2
  Logical Operator1/1 -> 2_val_shift_register/1
  Bus Selector/4 -> Unit Delay Enabled Resettable Synchronous8/3, Unit Delay Enabled Resettable Synchronous9/3, 2_val_shift_register/3  "<reset>"
  Logical Operator3/1 -> Logical Operator/2
  Logical Operator/1 -> Unit Delay Enabled Resettable Synchronous8/2, Unit Delay Enabled Resettable Synchronous9/2
  Switch/1 -> Unit Delay Enabled Resettable Synchronous8/1
  Logical Operator2/1 -> Switch1/2, Switch/2, Logical Operator/1
  Switch1/1 -> Unit Delay Enabled Resettable Synchronous9/1
  Unit Delay Enabled Resettable Synchronous9/1 -> Mux/1, dataOut/1
  Mux/1 -> state/1
  Unit Delay Enabled Resettable Synchronous8/1 -> Mux/2, Switch1/3

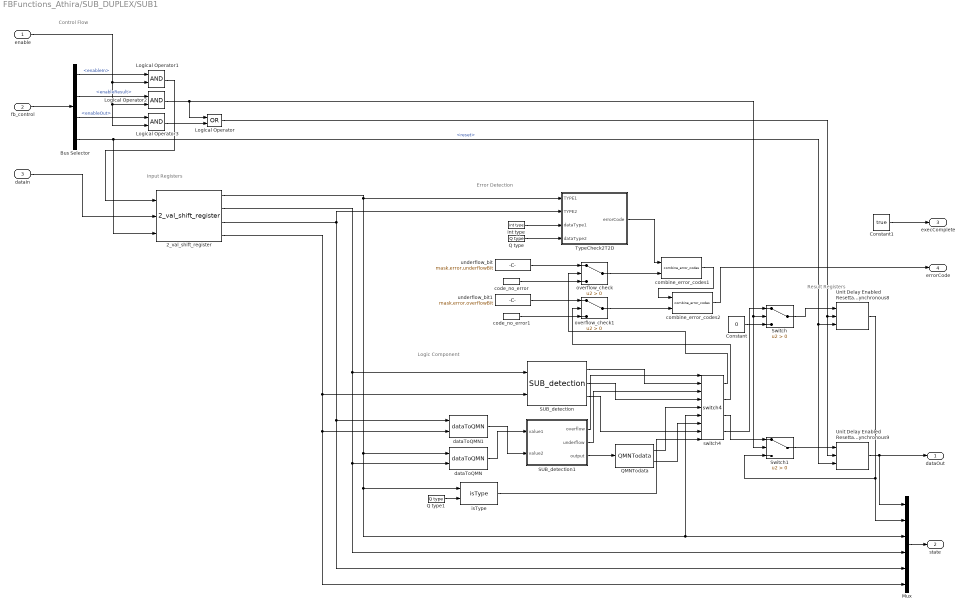
== system FBFunctions_Athira/SUB_DUPLEX/SUB1 ==
  note: Logic Component
  note: Input Registers
  note: Control Flow
  note: Error Detection
  note: Result Registers
  enable : Inport  OutDataTypeStr=boolean
  fb_control : Inport  Port=2  OutDataTypeStr=Bus: fb_control
  dataIn : Inport  Port=3  OutDataTypeStr=int32
  2_val_shift_register : library/2_val_shift_register  SystemSampleTime=-1
  Bus Selector : BusSelector  OutputSignals=enableIn,enableResult,enableOut,reset
  Constant : Constant  Value=0  OutDataTypeStr=int32
  Constant1 : Constant  Value=true  SampleTime=-1
  Logical Operator : Logic  Operator=OR  AllPortsSameDT=off  OutDataTypeStr=boolean
  Logical Operator1 : Logic  AllPortsSameDT=off  OutDataTypeStr=boolean
  Logical Operator2 : Logic  AllPortsSameDT=off  OutDataTypeStr=boolean
  Logical Operator3 : Logic  AllPortsSameDT=off  OutDataTypeStr=boolean
  Mux : Mux  Inputs=6
  Q type : library/Q type  SystemSampleTime=-1
  Q type1 : library/Q type  SystemSampleTime=-1
  QMNTodata : library/QMNTodata  SystemSampleTime=-1
      link override fractional2: lidx=31  ridx=24
  SUB_detection : library/SUB_detection  SystemSampleTime=-1
  SUB_detection1 : Subsystem  AncestorBlock=library/SUB_detection
  Switch : Switch  Criteria=u2 > Threshold
  Switch1 : Switch  Criteria=u2 > Threshold
  TypeCheck2T2D : Subsystem  AncestorBlock=library/TypeCheck2T2D
  Unit Delay Enabled Resettable Synchronous8 : hdlsllib/Discrete/Unit Delay Enabled Resettable Synchronous  InitialCondition=0.0  SampleTime=-1
      settings: SourceProductName=HDL Coder  SourceProductBaseCode=HD
  Unit Delay Enabled Resettable Synchronous9 : hdlsllib/Discrete/Unit Delay Enabled Resettable Synchronous  InitialCondition=0.0  SampleTime=-1
      settings: SourceProductName=HDL Coder  SourceProductBaseCode=HD
  code_no_error : library/code_no_error  SystemSampleTime=-1
  code_no_error1 : library/code_no_error  SystemSampleTime=-1
  combine_error_codes1 : library/combine_error_codes  SystemSampleTime=-1
  combine_error_codes2 : library/combine_error_codes  SystemSampleTime=-1
  dataToQMN : library/dataToQMN  SystemSampleTime=-1
  dataToQMN1 : library/dataToQMN  SystemSampleTime=-1
  int type : library/int type  SystemSampleTime=-1
  isType : library/isType  SystemSampleTime=-1
  overflow_check : Switch  Criteria=u2 > Threshold
  overflow_check1 : Switch  Criteria=u2 > Threshold
  switch4 : library/switch4  SystemSampleTime=-1
  underflow_bit : Constant  Value=mask.error.underflowBit  SampleTime=-1
  underflow_bit1 : Constant  Value=mask.error.overflowBit  SampleTime=-1
  dataOut : Outport
  state : Outport  Port=2
  execComplete : Outport  Port=3  OutDataTypeStr=boolean  PortDimensions=1
  errorCode : Outport  Port=4  PortDimensions=1
  wires:
  dataToQMN/1 -> SUB_detection1/1(value1)
  dataToQMN1/1 -> SUB_detection1/2(value2)
  switch4/1 -> overflow_check/2
  SUB_detection1/1(overflow) -> switch4/1
  QMNTodata/2 -> switch4/7
  2_val_shift_register/1 -> isType/1, Mux/3, switch4/6, dataToQMN/1, TypeCheck2T2D/1(TYPE1)
  SUB_detection/1 -> switch4/2
  isType/1 -> switch4/9
  SUB_detection/2 -> switch4/4
  Q type1/1 -> isType/2
  switch4/2 -> overflow_check1/2
  2_val_shift_register/4 -> Mux/6, dataToQMN1/2, SUB_detection/2
  SUB_detection1/2(underflow) -> switch4/3
  switch4/4 -> Switch/1
  SUB_detection1/3(output) -> QMNTodata/1
  switch4/3 -> Switch1/1
  2_val_shift_register/3 -> Mux/5, dataToQMN1/1, TypeCheck2T2D/2(TYPE2)
  2_val_shift_register/2 -> Mux/4, dataToQMN/2, SUB_detection/1
  QMNTodata/1 -> switch4/5
  SUB_detection/3 -> switch4/8
  combine_error_codes1/1 -> combine_error_codes2/1
  underflow_bit1/1 -> overflow_check1/1
  code_no_error1/1 -> overflow_check1/3
  overflow_check1/1 -> combine_error_codes2/2
  overflow_check/1 -> combine_error_codes1/2
  code_no_error/1 -> overflow_check/3
  underflow_bit/1 -> overflow_check/1
  combine_error_codes2/1 -> errorCode/1
  int type/1 -> TypeCheck2T2D/3(dataType1)
  Q type/1 -> TypeCheck2T2D/4(dataType2)
  TypeCheck2T2D/1(errorCode) -> combine_error_codes1/1
  enable/1 -> Logical Operator1/2, Logical Operator3/2, Logical Operator2/2
  Bus Selector/2 -> Logical Operator2/1  "<enableResult>"
  Bus Selector/1 -> Logical Operator1/1  "<enableIn>"
  Bus Selector/3 -> Logical Operator3/1  "<enableOut>"
  fb_control/1 -> Bus Selector/1
  Constant1/1 -> execComplete/1
  Constant/1 -> Switch/3
  dataIn/1 -> 2_val_shift_register/2
  Logical Operator1/1 -> 2_val_shift_register/1
  Bus Selector/4 -> Unit Delay Enabled Resettable Synchronous8/3, Unit Delay Enabled Resettable Synchronous9/3, 2_val_shift_register/3  "<reset>"
  Logical Operator3/1 -> Logical Operator/2
  Logical Operator/1 -> Unit Delay Enabled Resettable Synchronous8/2, Unit Delay Enabled Resettable Synchronous9/2
  Switch/1 -> Unit Delay Enabled Resettable Synchronous8/1
  Logical Operator2/1 -> Switch1/2, Switch/2, Logical Operator/1
  Switch1/1 -> Unit Delay Enabled Resettable Synchronous9/1
  Unit Delay Enabled Resettable Synchronous9/1 -> Mux/1, dataOut/1
  Mux/1 -> state/1
  Unit Delay Enabled Resettable Synchronous8/1 -> Mux/2, Switch1/3

== system FBFunctions_Athira/SUB_DUPLEX/State Comparator ==
  StateA : Inport  RequirementInfo={} %GIDa_850ba5fb_bec6_40a7_bff2_e88e25707b72
  StateB : Inport  RequirementInfo={} %GIDa_31d9701c_a33d_4ba1_b762_d6eba5e746ea  Port=2
  execComplete : Inport  RequirementInfo={} %GIDa_6900b5eb_6e34_4b5c_ab46_3bf84fbb4fde  Port=3
  Compare To Zero : simulink/Logic and Bit Operations/Compare To Zero  relop=>  OutDataTypeStr=boolean
  Constant1 : Constant  RequirementInfo={} %GIDa_e6dc7871_9460_47b7_844d_fe346f2ff008  Value=false  SampleTime=-1
  Relational Operator : RelationalOperator  RequirementInfo={} %GIDa_bc019a10_ee56_46ec_8d92_4f9a7b675e24  Operator=~=  OutDataTypeStr=boolean  RndMeth=Simplest
  Sum of Elements : Sum  RequirementInfo={} %GIDa_4b7ccedc_73e5_4206_ba44_2065d6a036fb  Inputs=+
  Switch1 : Switch  RequirementInfo={} %GIDa_a5db4cb6_7e1e_4dca_a520_beca643cf818  Criteria=u2 > Threshold
  stateError : Outport  RequirementInfo={} %GIDa_debaf768_048f_4ef3_86a7_3d4e6bd99aa3
  wires:
  Compare To Zero/1 -> Switch1/1
  Sum of Elements/1 -> Compare To Zero/1
  Relational Operator/1 -> Sum of Elements/1
  Switch1/1 -> stateError/1
  execComplete/1 -> Switch1/2
  Constant1/1 -> Switch1/3
  StateB/1 -> Relational Operator/2
  StateA/1 -> Relational Operator/1

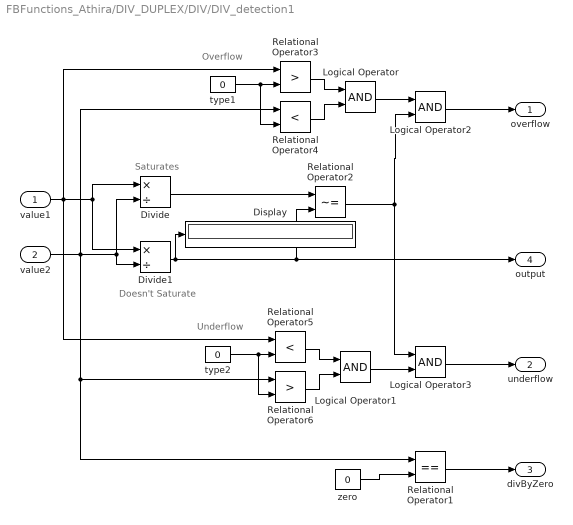
== system FBFunctions_Athira/DIV_DUPLEX/DIV/DIV_detection1 ==
  note: Underflow
  note: Overflow
  note: Doesn't Saturate
  note: Saturates
  value1 : Inport
  value2 : Inport  Port=2
  Display : Display
      settings: Format=long_e
  Divide : Product  Inputs=*/  SaturateOnIntegerOverflow=on
  Divide1 : Product  Inputs=*/
  Logical Operator{,1..3} (4 alike) : Logic  AllPortsSameDT=off  OutDataTypeStr=boolean
  Relational Operator1 : RelationalOperator  Operator===  OutDataTypeStr=boolean  RndMeth=Nearest
  Relational Operator2 : RelationalOperator  Operator=~=  OutDataTypeStr=boolean  RndMeth=Nearest
  Relational Operator3 : RelationalOperator  Operator=>  OutDataTypeStr=boolean  RndMeth=Nearest
  Relational Operator4 : RelationalOperator  Operator=<  OutDataTypeStr=boolean  RndMeth=Nearest
  Relational Operator5 : RelationalOperator  Operator=<  OutDataTypeStr=boolean  RndMeth=Nearest
  Relational Operator6 : RelationalOperator  Operator=>  OutDataTypeStr=boolean  RndMeth=Nearest
  type1 : Constant  Value=0  OutDataTypeStr=Inherit: Inherit via back propagation
  type2 : Constant  Value=0  OutDataTypeStr=Inherit: Inherit via back propagation
  zero : Constant  Value=0  OutDataTypeStr=Inherit: Inherit via back propagation  SampleTime=-1
  overflow : Outport  OutDataTypeStr=boolean  PortDimensions=1
  underflow : Outport  Port=2  OutDataTypeStr=boolean  PortDimensions=1
  divByZero : Outport  Port=3  OutDataTypeStr=boolean  PortDimensions=1
  output : Outport  Port=4  PortDimensions=1
  wires:
  Relational Operator1/1 -> divByZero/1
  zero/1 -> Relational Operator1/2
  Logical Operator3/1 -> underflow/1
  Logical Operator2/1 -> overflow/1
  Relational Operator2/1 -> Logical Operator2/2, Logical Operator3/1
  Logical Operator1/1 -> Logical Operator3/2
  Relational Operator5/1 -> Logical Operator1/1
  Relational Operator6/1 -> Logical Operator1/2
  Divide1/1 -> Relational Operator2/2, output/1, Display/1
  type2/1 -> Relational Operator5/2, Relational Operator6/2
  Divide/1 -> Relational Operator2/1
  Logical Operator/1 -> Logical Operator2/1
  Relational Operator4/1 -> Logical Operator/2
  Relational Operator3/1 -> Logical Operator/1
  type1/1 -> Relational Operator3/2, Relational Operator4/2
  value2/1 -> Divide/2, Divide1/2, Relational Operator4/1, Relational Operator6/1, Relational Operator1/1
  value1/1 -> Relational Operator3/1, Divide/1, Divide1/1, Relational Operator5/1

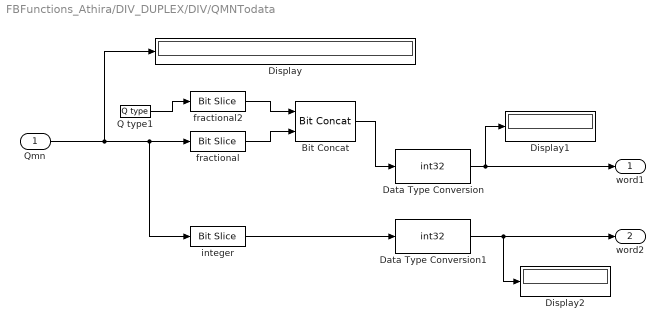
== system FBFunctions_Athira/DIV_DUPLEX/DIV/QMNTodata ==
  Qmn : Inport
  Bit Concat : hdlsllib/Logic and Bit Operations/Bit Concat  numInputs=2
      settings: SourceProductName=HDL Coder  SourceProductBaseCode=HD
  Data Type Conversion : DataTypeConversion  OutDataTypeStr=int32  ConvertRealWorld=Stored Integer (SI)
  Data Type Conversion1 : DataTypeConversion  OutDataTypeStr=int32  ConvertRealWorld=Stored Integer (SI)
  Display : Display
      settings: Format=long_e
  Display1 : Display
  Display2 : Display
  Q type1 : library/Q type  SystemSampleTime=-1
  fractional : hdlsllib/Logic and Bit Operations/Bit Slice  lidx=fractionalNumBits-1  ridx=0
  fractional2 : hdlsllib/Logic and Bit Operations/Bit Slice  lidx=31  ridx=24
  integer : hdlsllib/Logic and Bit Operations/Bit Slice  lidx=integerNumBits+fractionalNumBits-1  ridx=fractionalNumBits
  word1 : Outport  OutDataTypeStr=int32  PortDimensions=1
  word2 : Outport  Port=2  OutDataTypeStr=int32  PortDimensions=1
  wires:
  Bit Concat/1 -> Data Type Conversion/1
  fractional2/1 -> Bit Concat/1
  Q type1/1 -> fractional2/1
  fractional/1 -> Bit Concat/2
  integer/1 -> Data Type Conversion1/1
  Qmn/1 -> fractional/1, integer/1, Display/1
  Data Type Conversion1/1 -> word2/1, Display2/1
  Data Type Conversion/1 -> word1/1, Display1/1

== system FBFunctions_Athira/DIV_DUPLEX/DIV/dataToQMN ==
  word1 : Inport  OutDataTypeStr=int32
  word2 : Inport  Port=2  OutDataTypeStr=int32
  Bit Concat : hdlsllib/Logic and Bit Operations/Bit Concat  numInputs=2
      settings: SourceProductName=HDL Coder  SourceProductBaseCode=HD
  Data Type Conversion : DataTypeConversion  OutDataTypeStr=QType  ConvertRealWorld=Stored Integer (SI)
  Display : Display
      settings: Format=long_e
  fractional : hdlsllib/Logic and Bit Operations/Bit Slice  lidx=fractionalNumBits-1  ridx=0
  integer : hdlsllib/Logic and Bit Operations/Bit Slice  lidx=integerNumBits-1  ridx=0
  Qmn : Outport  OutDataTypeStr=QType  PortDimensions=1
  wires:
  Data Type Conversion/1 -> Qmn/1, Display/1
  Bit Concat/1 -> Data Type Conversion/1
  fractional/1 -> Bit Concat/2
  integer/1 -> Bit Concat/1
  word2/1 -> integer/1
  word1/1 -> fractional/1

== system FBFunctions_Athira/DIV_DUPLEX/DIV/dataToQMN1 ==
  word1 : Inport  OutDataTypeStr=int32
  word2 : Inport  Port=2  OutDataTypeStr=int32
  Bit Concat : hdlsllib/Logic and Bit Operations/Bit Concat  numInputs=2
      settings: SourceProductName=HDL Coder  SourceProductBaseCode=HD
  Data Type Conversion : DataTypeConversion  OutDataTypeStr=QType  ConvertRealWorld=Stored Integer (SI)
  Display : Display
      settings: Format=long_e
  fractional : hdlsllib/Logic and Bit Operations/Bit Slice  lidx=fractionalNumBits-1  ridx=0
  integer : hdlsllib/Logic and Bit Operations/Bit Slice  lidx=integerNumBits-1  ridx=0
  Qmn : Outport  OutDataTypeStr=QType  PortDimensions=1
  wires:
  Data Type Conversion/1 -> Qmn/1, Display/1
  Bit Concat/1 -> Data Type Conversion/1
  fractional/1 -> Bit Concat/2
  integer/1 -> Bit Concat/1
  word2/1 -> integer/1
  word1/1 -> fractional/1

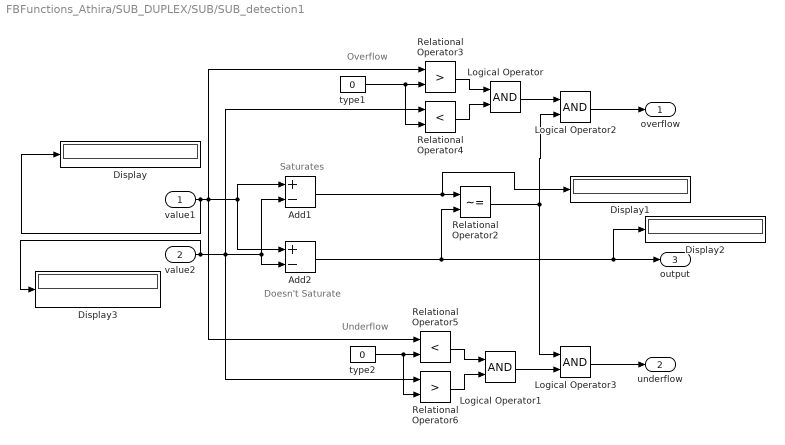
== system FBFunctions_Athira/SUB_DUPLEX/SUB/SUB_detection1 ==
  note: Underflow
  note: Overflow
  note: Doesn't Saturate
  note: Saturates
  value1 : Inport
  value2 : Inport  Port=2
  Add1 : Sum  Inputs=+-  SaturateOnIntegerOverflow=on
  Add2 : Sum  Inputs=+-
  Display{,1..3} (4 alike) : Display
      settings: Format=long_e
  Logical Operator{,1..3} (4 alike) : Logic  AllPortsSameDT=off  OutDataTypeStr=boolean
  Relational Operator2 : RelationalOperator  Operator=~=  OutDataTypeStr=boolean  RndMeth=Nearest
  Relational Operator3 : RelationalOperator  Operator=>  OutDataTypeStr=boolean  RndMeth=Nearest
  Relational Operator4 : RelationalOperator  Operator=<  OutDataTypeStr=boolean  RndMeth=Nearest
  Relational Operator5 : RelationalOperator  Operator=<  OutDataTypeStr=boolean  RndMeth=Nearest
  Relational Operator6 : RelationalOperator  Operator=>  OutDataTypeStr=boolean  RndMeth=Nearest
  type1 : Constant  Value=0  OutDataTypeStr=Inherit: Inherit via back propagation
  type2 : Constant  Value=0  OutDataTypeStr=Inherit: Inherit via back propagation
  overflow : Outport  OutDataTypeStr=boolean  PortDimensions=1
  underflow : Outport  Port=2  OutDataTypeStr=boolean  PortDimensions=1
  output : Outport  Port=3  PortDimensions=1
  wires:
  Logical Operator3/1 -> underflow/1
  Logical Operator2/1 -> overflow/1
  Relational Operator2/1 -> Logical Operator2/2, Logical Operator3/1
  Logical Operator1/1 -> Logical Operator3/2
  Relational Operator5/1 -> Logical Operator1/1
  Relational Operator6/1 -> Logical Operator1/2
  Add2/1 -> Relational Operator2/2, output/1, Display2/1
  type2/1 -> Relational Operator5/2, Relational Operator6/2
  Add1/1 -> Relational Operator2/1, Display1/1
  Logical Operator/1 -> Logical Operator2/1
  Relational Operator4/1 -> Logical Operator/2
  Relational Operator3/1 -> Logical Operator/1
  type1/1 -> Relational Operator3/2, Relational Operator4/2
  value2/1 -> Add1/2, Add2/2, Relational Operator4/1, Relational Operator6/1, Display3/1
  value1/1 -> Relational Operator3/1, Add2/1, Add1/1, Relational Operator5/1, Display/1

== system FBFunctions_Athira/SUB_DUPLEX/SUB/dataToQMN ==
  word1 : Inport  OutDataTypeStr=int32
  word2 : Inport  Port=2  OutDataTypeStr=int32
  Bit Concat : hdlsllib/Logic and Bit Operations/Bit Concat  numInputs=2
      settings: SourceProductName=HDL Coder  SourceProductBaseCode=HD
  Data Type Conversion : DataTypeConversion  OutDataTypeStr=QType  ConvertRealWorld=Stored Integer (SI)
  fractional : hdlsllib/Logic and Bit Operations/Bit Slice  lidx=fractionalNumBits-1  ridx=0
  integer : hdlsllib/Logic and Bit Operations/Bit Slice  lidx=integerNumBits-1  ridx=0
  Qmn : Outport  OutDataTypeStr=QType  PortDimensions=1
  wires:
  Data Type Conversion/1 -> Qmn/1
  Bit Concat/1 -> Data Type Conversion/1
  fractional/1 -> Bit Concat/2
  integer/1 -> Bit Concat/1
  word2/1 -> integer/1
  word1/1 -> fractional/1

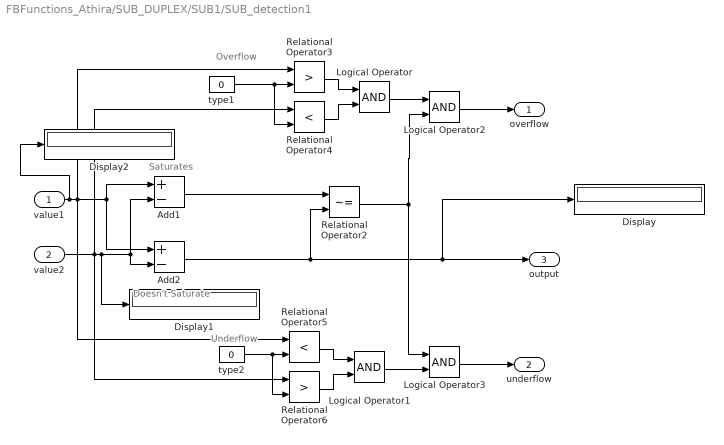
== system FBFunctions_Athira/SUB_DUPLEX/SUB1/SUB_detection1 ==
  note: Underflow
  note: Overflow
  note: Doesn't Saturate
  note: Saturates
  value1 : Inport
  value2 : Inport  Port=2
  Add1 : Sum  Inputs=+-  SaturateOnIntegerOverflow=on
  Add2 : Sum  Inputs=+-
  Display : Display
      settings: Format=long_e
  Display1 : Display
      settings: Format=long_e
  Display2 : Display
      settings: Format=long_e
  Logical Operator{,1..3} (4 alike) : Logic  AllPortsSameDT=off  OutDataTypeStr=boolean
  Relational Operator2 : RelationalOperator  Operator=~=  OutDataTypeStr=boolean  RndMeth=Nearest
  Relational Operator3 : RelationalOperator  Operator=>  OutDataTypeStr=boolean  RndMeth=Nearest
  Relational Operator4 : RelationalOperator  Operator=<  OutDataTypeStr=boolean  RndMeth=Nearest
  Relational Operator5 : RelationalOperator  Operator=<  OutDataTypeStr=boolean  RndMeth=Nearest
  Relational Operator6 : RelationalOperator  Operator=>  OutDataTypeStr=boolean  RndMeth=Nearest
  type1 : Constant  Value=0  OutDataTypeStr=Inherit: Inherit via back propagation
  type2 : Constant  Value=0  OutDataTypeStr=Inherit: Inherit via back propagation
  overflow : Outport  OutDataTypeStr=boolean  PortDimensions=1
  underflow : Outport  Port=2  OutDataTypeStr=boolean  PortDimensions=1
  output : Outport  Port=3  PortDimensions=1
  wires:
  Logical Operator3/1 -> underflow/1
  Logical Operator2/1 -> overflow/1
  Relational Operator2/1 -> Logical Operator2/2, Logical Operator3/1
  Logical Operator1/1 -> Logical Operator3/2
  Relational Operator5/1 -> Logical Operator1/1
  Relational Operator6/1 -> Logical Operator1/2
  Add2/1 -> Relational Operator2/2, output/1, Display/1
  type2/1 -> Relational Operator5/2, Relational Operator6/2
  Add1/1 -> Relational Operator2/1
  Logical Operator/1 -> Logical Operator2/1
  Relational Operator4/1 -> Logical Operator/2
  Relational Operator3/1 -> Logical Operator/1
  type1/1 -> Relational Operator3/2, Relational Operator4/2
  value2/1 -> Add1/2, Add2/2, Display1/1, Relational Operator4/1, Relational Operator6/1
  value1/1 -> Relational Operator3/1, Add2/1, Add1/1, Relational Operator5/1, Display2/1

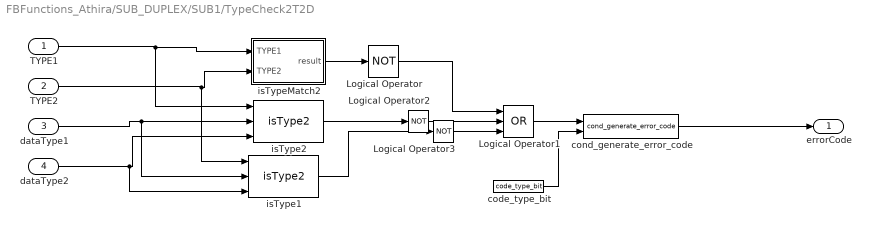
== system FBFunctions_Athira/SUB_DUPLEX/SUB1/TypeCheck2T2D ==
  TYPE1 : Inport
  TYPE2 : Inport  Port=2
  dataType1 : Inport  Port=3
  dataType2 : Inport  Port=4
  Logical Operator : Logic  Operator=NOT  AllPortsSameDT=off  OutDataTypeStr=boolean
  Logical Operator1 : Logic  Operator=OR  Inputs=3  AllPortsSameDT=off  OutDataTypeStr=boolean
  Logical Operator2 : Logic  Operator=NOT  Inputs=1  AllPortsSameDT=off  OutDataTypeStr=boolean
  Logical Operator3 : Logic  Operator=NOT  Inputs=1  AllPortsSameDT=off  OutDataTypeStr=boolean
  code_type_bit : library/code_type_bit  SystemSampleTime=-1
  cond_generate_error_code : library/cond_generate_error_code  SystemSampleTime=-1
  isType1 : library/isType2  SystemSampleTime=-1
  isType2 : library/isType2  SystemSampleTime=-1
  isTypeMatch2 : Subsystem  AncestorBlock=library/isTypeMatch2
  errorCode : Outport  OutDataTypeStr=uint32  PortDimensions=1
  wires:
  Logical Operator3/1 -> Logical Operator1/3
  Logical Operator2/1 -> Logical Operator1/2
  Logical Operator/1 -> Logical Operator1/1
  isTypeMatch2/1(result) -> Logical Operator/1
  Logical Operator1/1 -> cond_generate_error_code/1
  isType2/1 -> Logical Operator2/1
  isType1/1 -> Logical Operator3/1
  code_type_bit/1 -> cond_generate_error_code/2
  dataType2/1 -> isType2/3, isType1/3
  cond_generate_error_code/1 -> errorCode/1
  dataType1/1 -> isType2/2, isType1/2
  TYPE1/1 -> isType2/1, isTypeMatch2/1(TYPE1)
  TYPE2/1 -> isType1/1, isTypeMatch2/2(TYPE2)

== system FBFunctions_Athira/SUB_DUPLEX/SUB1/TypeCheck2T2D/isTypeMatch2 ==
  TYPE1 : Inport
  TYPE2 : Inport  Port=2
  Relational Operator1 : RelationalOperator  Operator===  RndMeth=Nearest
  typeMask : library/typeMask  SystemSampleTime=-1
      link override Apply Type Mask: BitMask=mask.typeBits
  typeMask1 : library/typeMask  SystemSampleTime=-1
  result : Outport  PortDimensions=1
  wires:
  typeMask1/1 -> Relational Operator1/2
  typeMask/1 -> Relational Operator1/1
  TYPE1/1 -> typeMask/1
  TYPE2/1 -> typeMask1/1
  Relational Operator1/1 -> result/1
